simulink library "orbit_data_bus"  (R2018b)
settings: Solver=VariableStepAuto  StartTime=0.0  StopTime=10.0  RelTol=1e-3
undefined symbols (not defined in the file): B_eci_T, dist_torque_Nm, eclipse, env_acc_mps2, sc2sun_eci_unit, simParams
settings Model: Creator=satcave1  LastModifiedBy=taylorreynolds

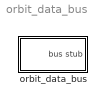
== system orbit_data_bus ==
  orbit_data_bus : Subsystem

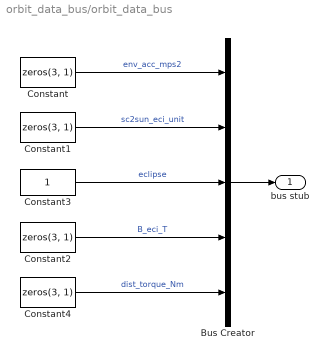
== system orbit_data_bus/orbit_data_bus ==
  Bus Creator : BusCreator  Inputs=env_acc_mps2,sc2sun_eci_unit,eclipse,B_eci_T,dist_torque_Nm  OutDataTypeStr=Bus: orbit_data
  Constant : Constant  Value=zeros(3, 1)  SampleTime=simParams.sample_time_s
  Constant1 : Constant  Value=zeros(3, 1)  SampleTime=simParams.sample_time_s
  Constant2 : Constant  Value=zeros(3, 1)  SampleTime=simParams.sample_time_s
  Constant3 : Constant  OutDataTypeStr=boolean
  Constant4 : Constant  Value=zeros(3, 1)  OutDataTypeStr=double  SampleTime=simParams.sample_time_s
  bus stub : Outport  OutDataTypeStr=Bus: orbit_data
  wires:
  Constant2/1 -> Bus Creator/4  "B_eci_T"
  Bus Creator/1 -> bus stub/1
  Constant/1 -> Bus Creator/1  "env_acc_mps2"
  Constant3/1 -> Bus Creator/3  "eclipse"
  Constant1/1 -> Bus Creator/2  "sc2sun_eci_unit"
  Constant4/1 -> Bus Creator/5  "dist_torque_Nm"
